simulink model "Gantry1DSimulinkV1"  (R2024b)
settings: Solver=FixedStepAuto  StartTime=0.0  StopTime=inf  FixedStep=0.05  RelTol=1e-3  EnableMultiTasking=on
libraries: raspberrypiBasiclib x5
settings Model: ExtModeTrigDuration=2  Creator=ioannisgeorgilas  LastModifiedBy=oskarchu
settings SolverCC: PositivePriorityOrder=on
settings OptimizationCC: EnhancedBackFolding=on  PassReuseOutputArgsAs=Individual arguments  ZeroExternalMemoryAtStartup=off  ZeroInternalMemoryAtStartup=off  MaxStackSize=200000  OptimizeBlockOrder=speed  DifferentSizesBufferReuse=on  OptimizationCustomize=off  EfficientTunableParamExpr=on
settings DebuggingCC: ParameterTunabilityLossMsg=error
settings HardwareCC: ProdBitPerPointer=32  ProdBitPerSizeT=32  ProdBitPerPtrDiffT=32  ProdLargestAtomicInteger=Long  ProdLargestAtomicFloat=Double  ProdWordSize=32  ProdLongLongMode=on  ProdHWDeviceType=ARM Compatible->ARM Cortex-A (32-bit)
settings RTWCC: Description=Embedded Coder  SystemTargetFile=ert.tlc  HardwareBoard=Raspberry Pi  TLCOptions="-aInlineSetEventsForThisBaseRateFcn=TLC_FALSE -aSuppressMultiTaskScheduler=TLC_FALSE  -aRateBasedStepFcn=0"  TemplateMakefile=ert_default_tmf  Toolchain=GNU GCC Embedded Linux  BuildConfiguration=Faster Runs
settings CodeAppCC: ForceParamTrailComments=on  IgnoreCustomStorageClasses=off  OperatorAnnotations=on  SimulinkDataObjDesc=on  SFDataObjDesc=on  InsertBlockDesc=on
settings ERTTargetCC: CodeReplacementLibrary=ARM Cortex-A CMSIS  SupportVariableSizeSignals=on  ExtModeTransport=2  ExtModeStaticAlloc=on  ExtModeMexFile=ext_xcp  ExtModeIntrfLevel=Level2 - Open  InlinedParameterPlacement=Hierarchical

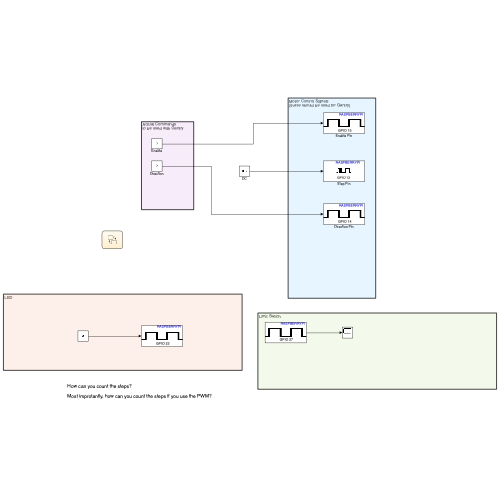
[thumbnail: Simulink's stored preview of the top-level diagram]
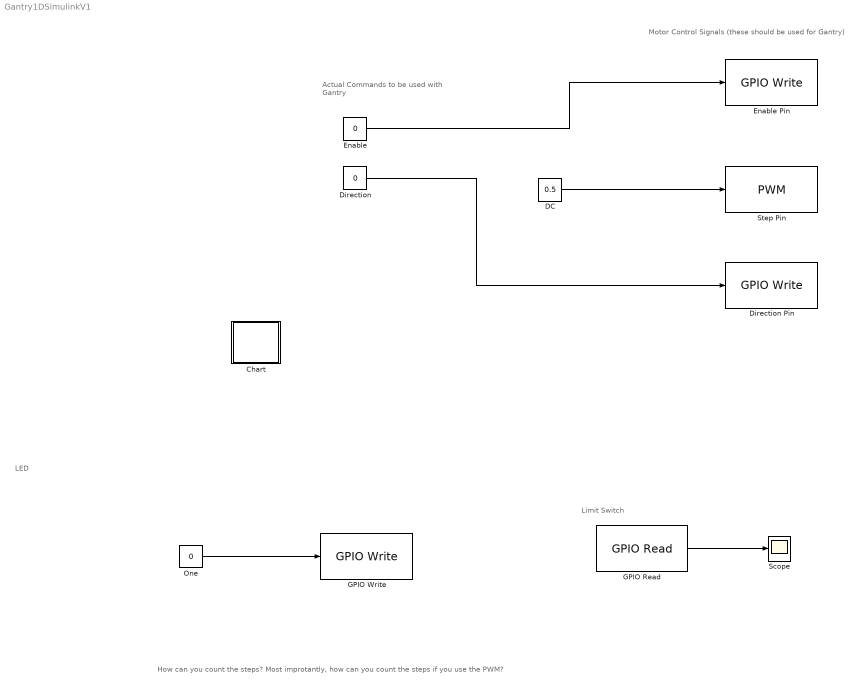
== system Gantry1DSimulinkV1 ==
  note: LED
  note: Actual Commands
      | to be used with Gantry
  note: How can you count the steps?
      |
      | Most improtantly, how can you count the steps if you use the PWM?
  note: Motor Control Signals
      | (these should be used for Gantry)
  note: Limit Switch
  Chart : Stateflow chart  TreatAsAtomicUnit=on
  DC : Constant  Value=0.5  SampleTime=-1
  Direction : Constant  Value=0  SampleTime=-1
  Direction Pin : raspberrypiBasiclib/GPIO Write  BoardProperty=Pi Zero 2 W  gpio=14  blockPlatform=Raspberry Pi  PinNumber=17  board=[]  direction=[]
  Enable : Constant  Value=0  SampleTime=-1
  Enable Pin : raspberrypiBasiclib/GPIO Write  BoardProperty=Pi Zero 2 W  gpio=15  blockPlatform=Raspberry Pi  PinNumber=17  board=[]  direction=[]
  GPIO Read : raspberrypiBasiclib/GPIO Read  BoardProperty=Pi Zero 2 W  gpio=27  SampleTime=-1  blockPlatform=Raspberry Pi  PinNumber=4  board=[]  direction=[]  internalResistor=[]
  GPIO Write : raspberrypiBasiclib/GPIO Write  BoardProperty=Pi Zero 2 W  gpio=22  blockPlatform=Raspberry Pi  PinNumber=17  board=[]  direction=[]
  One : Constant  Value=0  OutDataTypeStr=Inherit: Inherit via back propagation
  Scope : Scope
  Step Pin : raspberrypiBasiclib/PWM  board=Pi Zero W  Pin_=12  Frequency=200  blockPlatform=Raspberry Pi
  wires:
  Enable/1 -> Enable Pin/1
  Direction/1 -> Direction Pin/1
  DC/1 -> Step Pin/1
  GPIO Read/1 -> Scope/1
  One/1 -> GPIO Write/1

== stateflow chart Gantry1DSimulinkV1/Chart ==
